simulink model "roundingtest"  (Simulink 7.6)
settings: Solver=FixedStepDiscrete  StartTime=0.0  StopTime=10.0  FixedStep=1  RelTol=1e-3
settings Model: Creator=c2wt  LastModifiedBy=c2wt
settings DataIOCC: SaveFormat=Structure

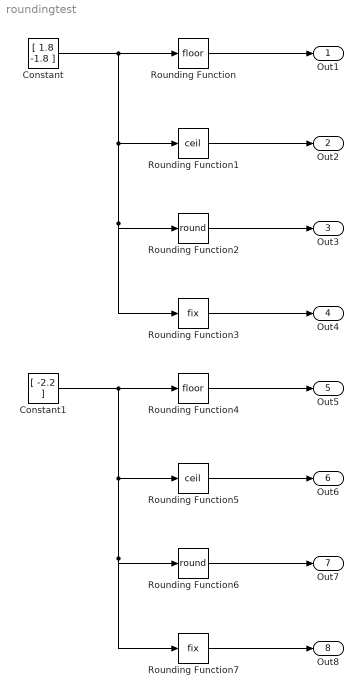
== system roundingtest ==
  Constant : Constant  Value=[ 1.8 -1.8 ]
  Constant1 : Constant  Value=[ -2.2 ]
  Rounding Function : Rounding
  Rounding Function1 : Rounding  Operator=ceil
  Rounding Function2 : Rounding  Operator=round
  Rounding Function3 : Rounding  Operator=fix
  Rounding Function4 : Rounding
  Rounding Function5 : Rounding  Operator=ceil
  Rounding Function6 : Rounding  Operator=round
  Rounding Function7 : Rounding  Operator=fix
  Out1 : Outport
  Out2 : Outport  Port=2
  Out3 : Outport  Port=3
  Out4 : Outport  Port=4
  Out5 : Outport  Port=5
  Out6 : Outport  Port=6
  Out7 : Outport  Port=7
  Out8 : Outport  Port=8
  wires:
  Constant/1 -> Rounding Function/1, Rounding Function1/1, Rounding Function2/1, Rounding Function3/1
  Rounding Function/1 -> Out1/1
  Rounding Function1/1 -> Out2/1
  Rounding Function2/1 -> Out3/1
  Rounding Function3/1 -> Out4/1
  Constant1/1 -> Rounding Function4/1, Rounding Function5/1, Rounding Function6/1, Rounding Function7/1
  Rounding Function4/1 -> Out5/1
  Rounding Function5/1 -> Out6/1
  Rounding Function6/1 -> Out7/1
  Rounding Function7/1 -> Out8/1
